simulink model "ComSerSimulink"  (R2018b)
settings: Solver=VariableStepAuto  StartTime=0.0  StopTime=100  RelTol=1e-3
undefined symbols (not defined in the file): serial
libraries: instrumentlib x4
settings Model: Creator=Admin  LastModifiedBy=Admin

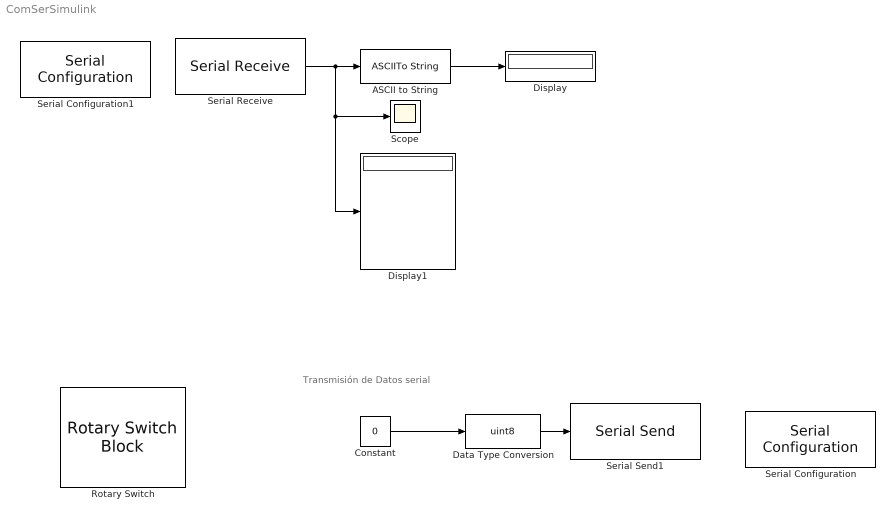
== system ComSerSimulink ==
  note: Transmisión de Datos serial
  ASCII to String : ASCIIToString
  Constant : Constant  Value=0
  Data Type Conversion : DataTypeConversion  OutDataTypeStr=uint8
  Display : Display
  Display1 : Display
  Rotary Switch : RotarySwitchBlock  WebBlockId=43
      settings: Values={{'Off', 'rojo', 'verde'}, [0 114 93]}
  Scope : Scope
  Serial Configuration : instrumentlib/Serial Configuration  Priority=-200000  ComPortMenu=COM7  ComPort=COM7  ObjConstructor=serial('COM7');  BaudRate=4800  DataBits=8  Parity=none  StopBits=1  FlowControl=none  Timeout=10  ByteOrder=LittleEndian
  Serial Configuration1 : instrumentlib/Serial Configuration  Priority=-200000  ComPortMenu=<Please select a port...>  ComPort=COM7  ObjConstructor=serial('COM7');  BaudRate=4800  DataBits=8  Parity=none  StopBits=1  FlowControl=none  Timeout=10  ByteOrder=LittleEndian
  Serial Receive : instrumentlib/Serial Receive  ComPortMenu=<Please select a port...>  ComPort=COM7  ObjConstructor=serial('COM7');  Terminator=<none>  DataSize=[1 1]  DataType=uint8  EnableBlockingMode=on  ActionDataUnavailable=Output last received value  CustomValue=0  SampleTime=0.01
  Serial Send1 : instrumentlib/Serial Send  ComPortMenu=COM7  ComPort=COM7  ObjConstructor=serial('COM7');  Terminator=<none>  EnableBlockingMode=on
  wires:
  Serial Receive/1 -> Scope/1, Display1/1, ASCII to String/1
  ASCII to String/1 -> Display/1
  Constant/1 -> Data Type Conversion/1
  Data Type Conversion/1 -> Serial Send1/1
